simulink model "frdm_lidar_servo"  (R2017a)
settings: Solver=VariableStepAuto  StartTime=0.0  StopTime=inf  RelTol=1e-3
libraries: frdmtfcshieldlib x1
settings Model: SimulationMode=external  Creator=WARA  LastModifiedBy=WARA

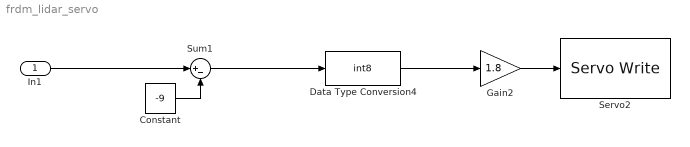
== system frdm_lidar_servo ==
  In1 : Inport
  Constant : Constant  Value=-9
  Data Type Conversion4 : DataTypeConversion  OutDataTypeStr=int8
  Gain2 : Gain  Gain=1.8
  Servo2 : frdmtfcshieldlib/Servo Write  WhichServo=1  minAngle=-30  maxAngle=70
      settings: SourceProductName=Simulink Coder Support Package for NXP FRDM-KL25Z Board  SourceProductBaseCode=EC_FREEDOM_BOARD
  Sum1 : Sum  Inputs=|+-
  wires:
  Sum1/1 -> Data Type Conversion4/1
  Constant/1 -> Sum1/2
  Data Type Conversion4/1 -> Gain2/1
  Gain2/1 -> Servo2/1
  In1/1 -> Sum1/1
